simulink model "gm_uz_resolver_mech_revolution_float"  (R2021a)
settings: Solver=FixedStepDiscrete  StartTime=0.0  StopTime=3/f_mech*resolver_polepairs*2  RelTol=1e-3
undefined symbols (not defined in the file or in its folder): bitToRpsFactor_16bit, f_mech, machine_polepairs, resolver_polepairs, t_ADC
libraries: hdlmdlgenlib x9, simulink x1
settings Model: Creator=micha  LastModifiedBy=micha
settings SolverCC: AlgebraicLoopSolver=TrustRegion
settings DataIOCC: LimitDataPoints=on  SaveOutput=off  SaveTime=off
settings OptimizationCC: BlockReduction=off  ConditionallyExecuteInputs=off  DefaultParameterBehavior=Inlined  LifeSpan=inf
settings DebuggingCC: AlgebraicLoopMsg=error  InheritedTsInSrcMsg=none  SingleTaskRateTransMsg=error  AllowSymbolicDim=off  StrictBusMsg=ErrorOnBusTreatedAsVector  SFUnexpectedBacktrackingDiag=warning  SFNoUnconditionalDefaultTransitionDiag=warning  SFExecutionAtInitializationDiag=none  SFMachineParentedDataDiag=warning  ArithmeticOperatorsInVariantConditions=warning
settings HardwareCC: ProdBitPerPointer=32  ProdBitPerSizeT=32  ProdBitPerPtrDiffT=32  ProdLargestAtomicFloat=None  ProdIntDivRoundTo=Undefined  ProdEndianess=Unspecified  ProdWordSize=32  ProdHWDeviceType=ASIC/FPGA->ASIC/FPGA  ProdEqTarget=off
settings SFSimCC: SimUseLocalCustomCode=off  CustomCodeUndefinedFunction=UseInterfaceOnly
settings RTWCC: RTWUseLocalCustomCode=off
settings CodeAppCC: StateflowObjectComments=on
settings GRTTargetCC: TargetLangStandard=C89/C90 (ANSI)
settings ConfigComp: CovScope=ReferencedModels  CovMetricSettings=dw  CovSaveCumulativeToWorkspaceVar=on  CovSaveSingleToWorkspaceVar=on  CovExternalEMLEnable=off  CovSFcnEnable=off

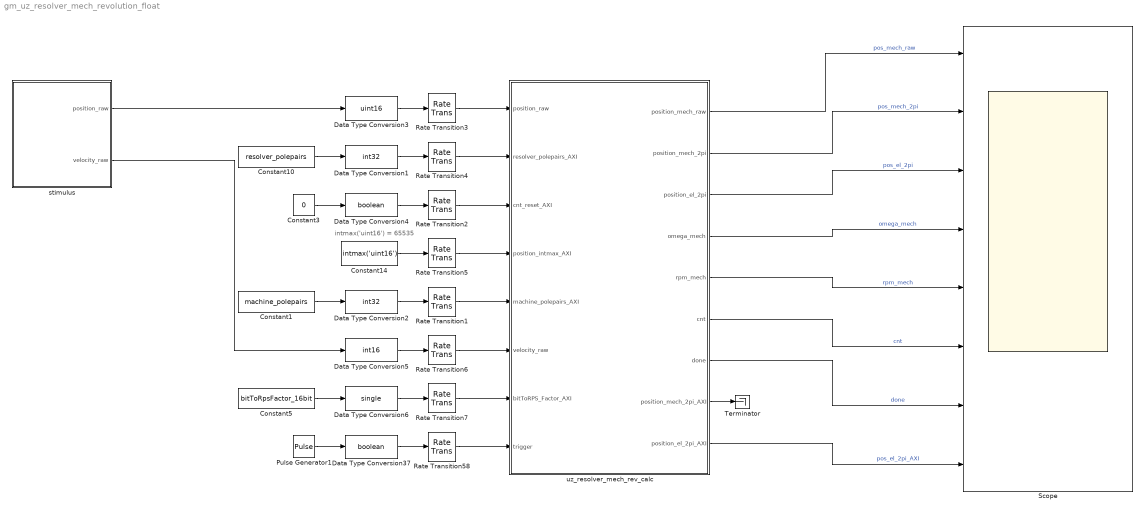
== system gm_uz_resolver_mech_revolution_float ==
  note: intmax('uint16') = 65535
  Constant1 : Constant  Value=machine_polepairs
  Constant10 : Constant  Value=resolver_polepairs
  Constant14 : Constant  Value=intmax('uint16')  OutDataTypeStr=int32  SampleTime=-1
  Constant3 : Constant  Value=0
  Constant5 : Constant  Value=bitToRpsFactor_16bit  SampleTime=-1
  Data Type Conversion1 : DataTypeConversion  OutDataTypeStr=int32
  Data Type Conversion2 : DataTypeConversion  OutDataTypeStr=int32
  Data Type Conversion3 : DataTypeConversion  OutDataTypeStr=uint16
  Data Type Conversion37 : DataTypeConversion  OutDataTypeStr=boolean
  Data Type Conversion4 : DataTypeConversion  OutDataTypeStr=boolean
  Data Type Conversion5 : DataTypeConversion  OutDataTypeStr=int16
  Data Type Conversion6 : DataTypeConversion  OutDataTypeStr=single
  Pulse Generator1 : DiscretePulseGenerator  PulseType=Time based  Period=t_ADC  PulseWidth=5
  Rate Transition{1..7,58} (8 alike) : RateTransition  OutPortSampleTime=t_clock
  Scope : Scope  NumInputPorts=8
  Terminator : Terminator
  stimulus : Subsystem
  uz_resolver_mech_rev_calc : Subsystem  TreatAsAtomicUnit=on
  wires:
  uz_resolver_mech_rev_calc/8(position_mech_2pi_AXI) -> Terminator/1
  uz_resolver_mech_rev_calc/9(position_el_2pi_AXI) -> Scope/8  "pos_el_2pi_AXI"
  uz_resolver_mech_rev_calc/5(rpm_mech) -> Scope/5  "rpm_mech"
  uz_resolver_mech_rev_calc/4(omega_mech) -> Scope/4  "omega_mech"
  Constant5/1 -> Data Type Conversion6/1
  Data Type Conversion6/1 -> Rate Transition7/1
  Rate Transition7/1 -> uz_resolver_mech_rev_calc/7(bitToRPS_Factor_AXI)
  stimulus/2(velocity_raw) -> Data Type Conversion5/1
  Rate Transition6/1 -> uz_resolver_mech_rev_calc/6(velocity_raw)
  Data Type Conversion5/1 -> Rate Transition6/1
  uz_resolver_mech_rev_calc/3(position_el_2pi) -> Scope/3  "pos_el_2pi"
  Rate Transition1/1 -> uz_resolver_mech_rev_calc/5(machine_polepairs_AXI)
  Constant1/1 -> Data Type Conversion2/1
  Data Type Conversion2/1 -> Rate Transition1/1
  stimulus/1(position_raw) -> Data Type Conversion3/1
  uz_resolver_mech_rev_calc/7(done) -> Scope/7  "done"
  uz_resolver_mech_rev_calc/6(cnt) -> Scope/6  "cnt"
  uz_resolver_mech_rev_calc/2(position_mech_2pi) -> Scope/2  "pos_mech_2pi"
  uz_resolver_mech_rev_calc/1(position_mech_raw) -> Scope/1  "pos_mech_raw"
  Data Type Conversion1/1 -> Rate Transition4/1
  Constant10/1 -> Data Type Conversion1/1
  Data Type Conversion3/1 -> Rate Transition3/1
  Rate Transition5/1 -> uz_resolver_mech_rev_calc/4(position_intmax_AXI)
  Constant14/1 -> Rate Transition5/1
  Rate Transition2/1 -> uz_resolver_mech_rev_calc/3(cnt_reset_AXI)
  Rate Transition3/1 -> uz_resolver_mech_rev_calc/1(position_raw)
  Rate Transition4/1 -> uz_resolver_mech_rev_calc/2(resolver_polepairs_AXI)
  Pulse Generator1/1 -> Data Type Conversion37/1
  Data Type Conversion37/1 -> Rate Transition58/1
  Data Type Conversion4/1 -> Rate Transition2/1
  Rate Transition58/1 -> uz_resolver_mech_rev_calc/8(trigger)
  Constant3/1 -> Data Type Conversion4/1

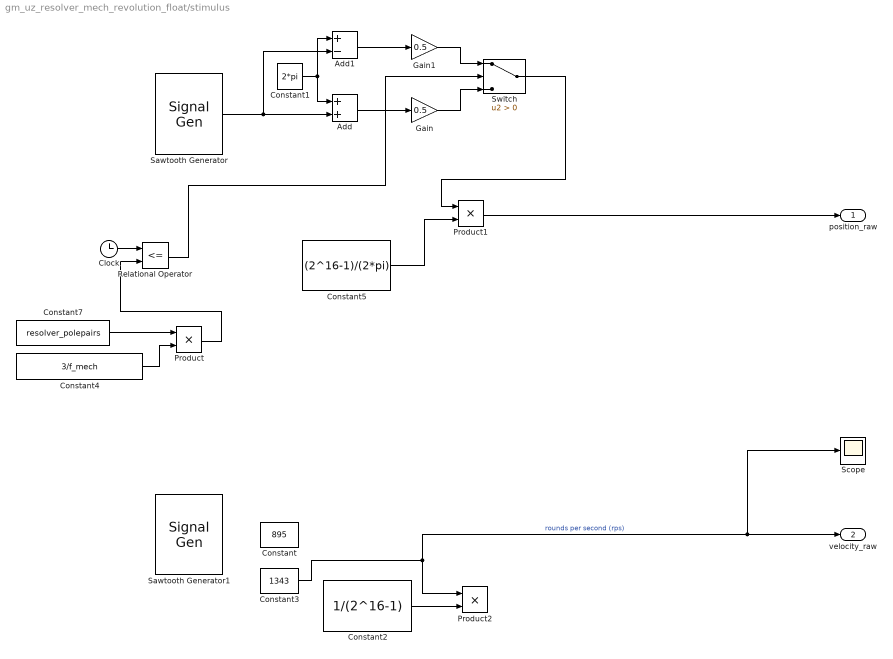
== system gm_uz_resolver_mech_revolution_float/stimulus ==
  Add : Sum
  Add1 : Sum  Inputs=+-
  Clock : Clock
  Constant : Constant  Value=895  SampleTime=-1
  Constant1 : Constant  Value=2*pi
  Constant2 : Constant  Value=1/(2^16-1)
  Constant3 : Constant  Value=1343  SampleTime=-1
  Constant4 : Constant  Value=3/f_mech
  Constant5 : Constant  Value=(2^16-1)/(2*pi)
  Constant7 : Constant  Value=resolver_polepairs
  Gain : Gain  Gain=0.5
  Gain1 : Gain  Gain=0.5
  Product : Product
  Product1 : Product
  Product2 : Product
  Relational Operator : RelationalOperator  Operator=<=  OutDataTypeStr=boolean  RndMeth=Simplest
  Sawtooth Generator : SignalGenerator  WaveForm=sawtooth  Amplitude=2*pi  Frequency=2*pi*f_mech  Units=rad/sec
  Sawtooth Generator1 : SignalGenerator  WaveForm=sawtooth  Frequency=2*pi*f_mech  Units=rad/sec
  Scope : Scope
  Switch : Switch  Criteria=u2 > Threshold
  position_raw : Outport
  velocity_raw : Outport  Port=2
  wires:
  Constant3/1 -> Product2/1, velocity_raw/1, Scope/1  "rounds per second (rps)"
  Constant2/1 -> Product2/2
  Product1/1 -> position_raw/1
  Relational Operator/1 -> Switch/2
  Constant7/1 -> Product/1
  Add/1 -> Gain/1
  Constant1/1 -> Add1/1, Add/1
  Gain1/1 -> Switch/1
  Add1/1 -> Gain1/1
  Switch/1 -> Product1/1
  Product/1 -> Relational Operator/2
  Constant5/1 -> Product1/2
  Gain/1 -> Switch/3
  Clock/1 -> Relational Operator/1
  Constant4/1 -> Product/2
  Sawtooth Generator/1 -> Add/2, Add1/2

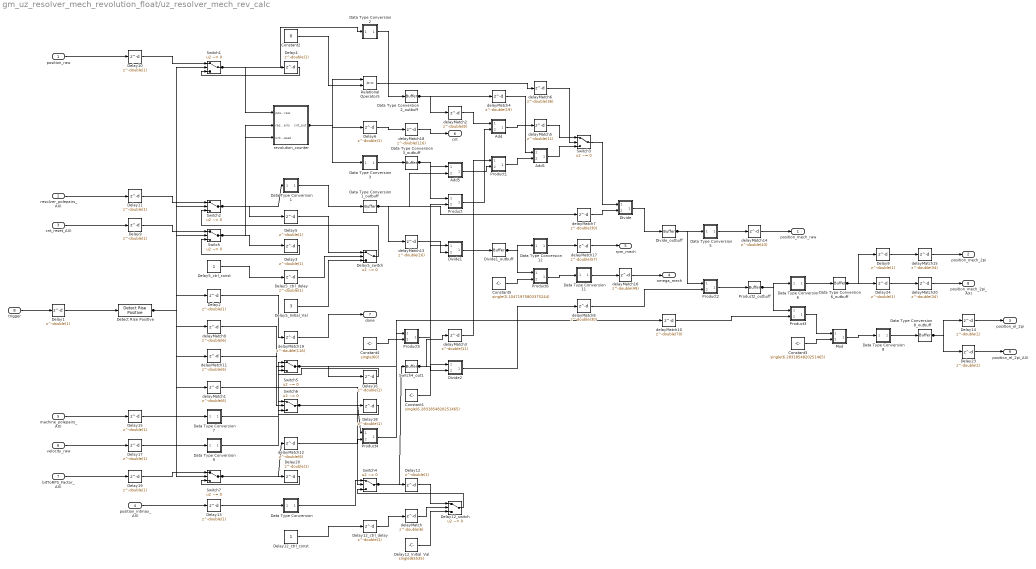
== system gm_uz_resolver_mech_revolution_float/uz_resolver_mech_rev_calc ==
  position_raw : Inport  OutDataTypeStr=uint16  PortDimensions=1  SampleTime=1e-08
  resolver_polepairs_AXI : Inport  Port=2  OutDataTypeStr=int32  PortDimensions=1  SampleTime=1e-08
  cnt_reset_AXI : Inport  Port=3  OutDataTypeStr=boolean  PortDimensions=1  SampleTime=1e-08
  position_intmax_AXI : Inport  Port=4  OutDataTypeStr=int32  PortDimensions=1  SampleTime=1e-08
  machine_polepairs_AXI : Inport  Port=5  OutDataTypeStr=int32  PortDimensions=1  SampleTime=1e-08
  velocity_raw : Inport  Port=6  OutDataTypeStr=int16  PortDimensions=1  SampleTime=1e-08
  bitToRPS_Factor_AXI : Inport  Port=7  OutDataTypeStr=single  PortDimensions=1  SampleTime=1e-08
  trigger : Inport  Port=8  OutDataTypeStr=boolean  PortDimensions=1  SampleTime=1e-08
  Add : Subsystem
      mask Display: disp('NFP\nadd');
  Add1 : Subsystem
      mask Display: disp('NFP\nadd');
  Add5 : Subsystem
      mask Display: disp('NFP\nadd');
  Constant1 : Constant  Value=single(6.2831854820251465)  OutDataTypeStr=single  SampleTime=1e-08
  Constant2 : Constant  Value=0  OutDataTypeStr=int16  SampleTime=1e-08
  Constant3 : Constant  Value=single(6.2831854820251465)  OutDataTypeStr=single  SampleTime=1e-08
  Constant4 : Constant  Value=single(60)  OutDataTypeStr=single  SampleTime=1e-08
  Constant5 : Constant  Value=single(0.10471975803375244)  OutDataTypeStr=single  SampleTime=1e-08
  Data Type Conversion : Subsystem
      mask Display: disp('NFP\nconv');
  Data Type Conversion1 : Subsystem
      mask Display: disp('NFP\nconv');
  Data Type Conversion11 : Subsystem
      mask Display: disp('NFP\nconv');
  Data Type Conversion12 : Subsystem
      mask Display: disp('NFP\nconv');
  Data Type Conversion1_outbuff : hdlmdlgenlib/Buffer
      settings: SourceProductBaseCode=SL
  Data Type Conversion2 : Subsystem
      mask Display: disp('NFP\nconv');
  Data Type Conversion2_outbuff : hdlmdlgenlib/Buffer
      settings: SourceProductBaseCode=SL
  Data Type Conversion3 : Subsystem
      mask Display: disp('NFP\nconv');
  Data Type Conversion3_outbuff : hdlmdlgenlib/Buffer
      settings: SourceProductBaseCode=SL
  Data Type Conversion5 : Subsystem
      mask Display: disp('NFP\nconv');
  Data Type Conversion6 : Subsystem
      mask Display: disp('NFP\nconv');
  Data Type Conversion6_outbuff : hdlmdlgenlib/Buffer
      settings: SourceProductBaseCode=SL
  Data Type Conversion7 : Subsystem
      mask Display: disp('NFP\nconv');
  Data Type Conversion8 : Subsystem
      mask Display: disp('NFP\nconv');
  Data Type Conversion8_outbuff : hdlmdlgenlib/Buffer
      settings: SourceProductBaseCode=SL
  Data Type Conversion9 : Subsystem
      mask Display: disp('NFP\nconv');
  Delay{1..6,8..20,23..24} (21 alike) : Delay  DelayLength=double(1)  InitialCondition=0  SampleTime=1e-08
  Delay12_Initial_Val : Constant  Value=single(65535)  OutDataTypeStr=single  SampleTime=1e-08
  Delay12_ctrl_const : Constant  OutDataTypeStr=boolean  SampleTime=1e-08
  Delay12_ctrl_delay : Delay  DelayLength=double(1)  InitialCondition=0  SampleTime=1e-08
  Delay12_switch : Switch  Criteria=u2 ~= 0  Threshold=double(0)  OutDataTypeStr=single  SampleTime=1e-08
  Delay5_Initial_Val : Constant  Value=3  OutDataTypeStr=int32  SampleTime=1e-08
  Delay5_ctrl_const : Constant  OutDataTypeStr=boolean  SampleTime=1e-08
  Delay5_ctrl_delay : Delay  DelayLength=double(1)  InitialCondition=0  SampleTime=1e-08
  Delay5_switch : Switch  Criteria=u2 ~= 0  Threshold=double(0)  OutDataTypeStr=int32  SampleTime=1e-08
  Detect Rise Positive : simulink/Logic and Bit Operations/Detect Rise Positive  vinit=0  OutDataTypeStr=boolean
  Divide : Subsystem
      mask Display: disp('NFP\nmul');
  Divide1 : Subsystem
      mask Display: disp('NFP\nmul');
  Divide1_outbuff : hdlmdlgenlib/Buffer
      settings: SourceProductBaseCode=SL
  Divide2 : Subsystem
      mask Display: disp('NFP\nmul');
  Divide_outbuff : hdlmdlgenlib/Buffer
      settings: SourceProductBaseCode=SL
  Mod : Subsystem
      mask Display: disp('NFP\nmath2');
  Product : Subsystem
      mask Display: disp('NFP\nmul');
  Product1 : Subsystem
      mask Display: disp('NFP\nmul');
  Product2 : Subsystem
      mask Display: disp('NFP\nmul');
  Product2_outbuff : hdlmdlgenlib/Buffer
      settings: SourceProductBaseCode=SL
  Product3 : Subsystem
      mask Display: disp('NFP\nmul');
  Product4 : Subsystem
      mask Display: disp('NFP\nmul');
  Product5 : Subsystem
      mask Display: disp('NFP\nmul');
  Product6 : Subsystem
      mask Display: disp('NFP\nmul');
  Relational Operator5 : RelationalOperator  OutDataTypeStr=boolean  SampleTime=1e-08  RndMeth=Nearest
  Switch : Switch  Criteria=u2 ~= 0  Threshold=double(0)  OutDataTypeStr=boolean  SampleTime=1e-08
  Switch1 : Switch  Criteria=u2 ~= 0  Threshold=double(0)  OutDataTypeStr=uint16  SampleTime=1e-08
  Switch2 : Switch  Criteria=u2 ~= 0  Threshold=double(0)  OutDataTypeStr=int32  SampleTime=1e-08
  Switch{3..7} (5 alike) : Switch  Criteria=u2 ~= 0  Threshold=double(0)  OutDataTypeStr=single  SampleTime=1e-08
  Switch4_out1 : hdlmdlgenlib/Buffer
      settings: SourceProductBaseCode=SL
  delayMatch{,1,9,11..12} (5 alike) : Delay  DelayLength=double(6)  InitialCondition=0  SampleTime=1e-08
  delayMatch10 : Delay  DelayLength=double(70)  InitialCondition=0  SampleTime=1e-08
  delayMatch13 : Delay  DelayLength=double(16)  InitialCondition=0  SampleTime=1e-08
  delayMatch14 : Delay  DelayLength=double(43)  InitialCondition=0  SampleTime=1e-08
  delayMatch15 : Delay  DelayLength=double(34)  InitialCondition=0  SampleTime=1e-08
  delayMatch16 : Delay  DelayLength=double(49)  InitialCondition=0  SampleTime=1e-08
  delayMatch17 : Delay  DelayLength=double(57)  InitialCondition=0  SampleTime=1e-08
  delayMatch18 : Delay  DelayLength=double(116)  InitialCondition=0  SampleTime=1e-08
  delayMatch19 : Delay  DelayLength=double(116)  InitialCondition=0  SampleTime=1e-08
  delayMatch2 : Delay  DelayLength=double(8)  InitialCondition=0  SampleTime=1e-08
  delayMatch20 : Delay  DelayLength=double(34)  InitialCondition=0  SampleTime=1e-08
  delayMatch3 : Delay  DelayLength=double(11)  InitialCondition=0  SampleTime=1e-08
  delayMatch4 : Delay  DelayLength=double(19)  InitialCondition=0  SampleTime=1e-08
  delayMatch5 : Delay  DelayLength=double(11)  InitialCondition=0  SampleTime=1e-08
  delayMatch6 : Delay  DelayLength=double(36)  InitialCondition=0  SampleTime=1e-08
  delayMatch7 : Delay  DelayLength=double(30)  InitialCondition=0  SampleTime=1e-08
  delayMatch8 : Delay  DelayLength=double(30)  InitialCondition=0  SampleTime=1e-08
  revolution_counter : Subsystem
  position_mech_raw : Outport  SampleTime=1e-08  VectorParamsAs1DForOutWhenUnconnected=off
  position_mech_2pi : Outport  Port=2  SampleTime=1e-08  VectorParamsAs1DForOutWhenUnconnected=off
  position_el_2pi : Outport  Port=3  SampleTime=1e-08  VectorParamsAs1DForOutWhenUnconnected=off
  omega_mech : Outport  Port=4  SampleTime=1e-08  VectorParamsAs1DForOutWhenUnconnected=off
  rpm_mech : Outport  Port=5  SampleTime=1e-08  VectorParamsAs1DForOutWhenUnconnected=off
  cnt : Outport  Port=6  SampleTime=1e-08  VectorParamsAs1DForOutWhenUnconnected=off
  done : Outport  Port=7  SampleTime=1e-08  VectorParamsAs1DForOutWhenUnconnected=off
  position_mech_2pi_AXI : Outport  Port=8  SampleTime=1e-08  VectorParamsAs1DForOutWhenUnconnected=off
  position_el_2pi_AXI : Outport  Port=9  SampleTime=1e-08  VectorParamsAs1DForOutWhenUnconnected=off
  wires:
  position_raw/1 -> Delay10/1
  resolver_polepairs_AXI/1 -> Delay11/1
  cnt_reset_AXI/1 -> Delay9/1
  position_intmax_AXI/1 -> Delay13/1
  machine_polepairs_AXI/1 -> Delay15/1
  velocity_raw/1 -> Delay17/1
  bitToRPS_Factor_AXI/1 -> Delay19/1
  trigger/1 -> Delay1/1
  delayMatch5/1 -> Switch3/1
  Constant1/1 -> Divide2/1(In1)
  Constant2/1 -> Relational Operator5/2
  Constant3/1 -> Mod/2(In2)
  Constant4/1 -> Product5/2(In2)
  Constant5/1 -> Product6/2(In2)
  delayMatch7/1 -> Divide/2(In2)
  delayMatch16/1 -> omega_mech/1
  delayMatch17/1 -> rpm_mech/1
  delayMatch2/1 -> Add/1(In1)
  Data Type Conversion3_outbuff/1 -> Product/1(In1), Add5/1(In1)
  delayMatch14/1 -> position_mech_raw/1
  Data Type Conversion6_outbuff/1 -> Delay8/1, Delay24/1
  Data Type Conversion8_outbuff/1 -> Delay23/1, Delay14/1
  Delay1/1 -> Detect Rise Positive/1
  Delay10/1 -> Switch1/1
  Delay11/1 -> Switch2/1
  Delay13/1 -> Data Type Conversion/1(In1)
  Delay14/1 -> position_el_2pi/1
  Delay15/1 -> Data Type Conversion7/1(In1)
  Delay17/1 -> Data Type Conversion9/1(In1)
  Delay19/1 -> Switch7/1
  delayMatch19/1 -> done/1
  Delay23/1 -> position_el_2pi_AXI/1
  delayMatch20/1 -> position_mech_2pi_AXI/1
  delayMatch18/1 -> cnt/1
  delayMatch15/1 -> position_mech_2pi/1
  Delay9/1 -> Switch/1
  delayMatch1/1 -> Switch4/2
  Divide_outbuff/1 -> Product2/1(In1), Data Type Conversion5/1(In1)
  Divide1_outbuff/1 -> Product6/1(In1), Data Type Conversion12/1(In1)
  delayMatch8/1 -> Product2/2(In2)
  Product2_outbuff/1 -> Product3/1(In1), Data Type Conversion6/1(In1)
  delayMatch6/1 -> Switch3/2
  Switch/1 -> revolution_counter/3(cnt_reset), Delay3/1
  Switch1/1 -> Data Type Conversion2/1(In1), revolution_counter/1(position_raw), Delay4/1
  Switch2/1 -> Data Type Conversion1/1(In1), revolution_counter/2(resolver_polepairs), Delay5/1
  Switch3/1 -> Divide/1(In1)
  delayMatch3/1 -> Product1/1(In1)
  delayMatch10/1 -> Product3/2(In2)
  delayMatch12/1 -> Product4/2(In2)
  revolution_counter/1(cnt_out) -> Data Type Conversion3/1(In1), Relational Operator5/1, Delay6/1
  Delay12_Initial_Val/1 -> Delay12_switch/3
  Delay12_ctrl_const/1 -> Delay12_ctrl_delay/1
  delayMatch/1 -> Delay12_switch/2
  Delay5_Initial_Val/1 -> Delay5_switch/3
  Delay5_ctrl_const/1 -> Delay5_ctrl_delay/1
  Delay5_ctrl_delay/1 -> Delay5_switch/2
  Add/1(Out1) -> delayMatch5/1
  Add1/1(Out1) -> Switch3/3
  Add5/1(Out1) -> Product1/2(In2)
  Data Type Conversion/1(Out1) -> Switch4/1
  Data Type Conversion1/1(Out1) -> Data Type Conversion1_outbuff/1
  Data Type Conversion11/1(Out1) -> delayMatch16/1
  Data Type Conversion12/1(Out1) -> delayMatch17/1
  Data Type Conversion2/1(Out1) -> Data Type Conversion2_outbuff/1
  Data Type Conversion3/1(Out1) -> Data Type Conversion3_outbuff/1
  Data Type Conversion5/1(Out1) -> delayMatch14/1
  Data Type Conversion6/1(Out1) -> Data Type Conversion6_outbuff/1
  Data Type Conversion7/1(Out1) -> Switch5/1
  Data Type Conversion8/1(Out1) -> Data Type Conversion8_outbuff/1
  Data Type Conversion9/1(Out1) -> Switch6/1
  Divide/1(Out1) -> Divide_outbuff/1
  Divide1/1(Out1) -> Divide1_outbuff/1
  Divide2/1(Out1) -> delayMatch8/1
  Mod/1(Out1) -> Data Type Conversion8/1(In1)
  Product/1(Out1) -> Add/2(In2)
  Product1/1(Out1) -> Add1/2(In2)
  Product2/1(Out1) -> Product2_outbuff/1
  Product3/1(Out1) -> Mod/1(In1)
  Product4/1(Out1) -> Product5/1(In1)
  Product5/1(Out1) -> Divide1/1(In1)
  Product6/1(Out1) -> Data Type Conversion11/1(In1)
  Delay12_ctrl_delay/1 -> delayMatch/1
  delayMatch9/1 -> Switch5/2
  delayMatch4/1 -> Add1/1(In1)
  Switch4_out1/1 -> delayMatch3/1, Product/2(In2), Divide2/2(In2)
  Data Type Conversion2_outbuff/1 -> delayMatch4/1, delayMatch2/1
  Relational Operator5/1 -> delayMatch6/1
  delayMatch13/1 -> Divide1/2(In2)
  delayMatch11/1 -> Switch6/2
  Detect Rise Positive/1 -> delayMatch11/1, delayMatch9/1, delayMatch1/1, Delay2/1, Switch1/2, Switch2/2, Switch/2, Switch7/2
  Switch7/1 -> delayMatch12/1, Delay20/1
  Data Type Conversion1_outbuff/1 -> delayMatch13/1, delayMatch7/1, Add5/2(In2)
  Delay8/1 -> delayMatch15/1
  Delay6/1 -> delayMatch18/1
  Delay2/1 -> delayMatch19/1
  Delay24/1 -> delayMatch20/1
  Switch4/1 -> Switch4_out1/1, Delay12/1
  Switch5/1 -> delayMatch10/1, Delay16/1
  Switch6/1 -> Product4/1(In1), Delay18/1
  Delay4/1 -> Switch1/3
  Delay5/1 -> Delay5_switch/1
  Delay5_switch/1 -> Switch2/3
  Delay3/1 -> Switch/3
  Delay12/1 -> Delay12_switch/1
  Delay12_switch/1 -> Switch4/3
  Delay16/1 -> Switch5/3
  Delay18/1 -> Switch6/3
  Delay20/1 -> Switch7/3

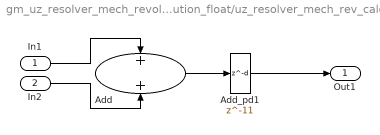
== system gm_uz_resolver_mech_revolution_float/uz_resolver_mech_rev_calc/Add ==
  In1 : Inport
  In2 : Inport  Port=2
  Add : Sum  OutDataTypeStr=single  SampleTime=1e-08
  Add_pd1 : Delay  DelayLength=11
  Out1 : Outport
  wires:
  In1/1 -> Add/1
  In2/1 -> Add/2
  Add/1 -> Add_pd1/1
  Add_pd1/1 -> Out1/1

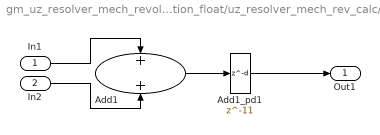
== system gm_uz_resolver_mech_revolution_float/uz_resolver_mech_rev_calc/Add1 ==
  In1 : Inport
  In2 : Inport  Port=2
  Add1 : Sum  OutDataTypeStr=single  SampleTime=1e-08
  Add1_pd1 : Delay  DelayLength=11
  Out1 : Outport
  wires:
  In1/1 -> Add1/1
  In2/1 -> Add1/2
  Add1/1 -> Add1_pd1/1
  Add1_pd1/1 -> Out1/1

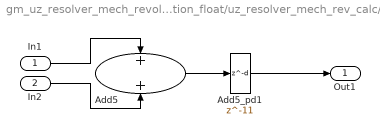
== system gm_uz_resolver_mech_revolution_float/uz_resolver_mech_rev_calc/Add5 ==
  In1 : Inport
  In2 : Inport  Port=2
  Add5 : Sum  OutDataTypeStr=single  SampleTime=1e-08
  Add5_pd1 : Delay  DelayLength=11
  Out1 : Outport
  wires:
  In1/1 -> Add5/1
  In2/1 -> Add5/2
  Add5/1 -> Add5_pd1/1
  Add5_pd1/1 -> Out1/1

== system gm_uz_resolver_mech_revolution_float/uz_resolver_mech_rev_calc/Data Type Conversion ==
  In1 : Inport
  Data Type Conversion : DataTypeConversion  OutDataTypeStr=single  SampleTime=1e-08
  Data Type Conversion_pd1 : Delay  DelayLength=6
  Out1 : Outport
  wires:
  In1/1 -> Data Type Conversion/1
  Data Type Conversion/1 -> Data Type Conversion_pd1/1
  Data Type Conversion_pd1/1 -> Out1/1

== system gm_uz_resolver_mech_revolution_float/uz_resolver_mech_rev_calc/Data Type Conversion1 ==
  In1 : Inport
  Data Type Conversion1 : DataTypeConversion  OutDataTypeStr=single  SampleTime=1e-08
  Data Type Conversion1_pd1 : Delay  DelayLength=6
  Out1 : Outport
  wires:
  In1/1 -> Data Type Conversion1/1
  Data Type Conversion1/1 -> Data Type Conversion1_pd1/1
  Data Type Conversion1_pd1/1 -> Out1/1

== system gm_uz_resolver_mech_revolution_float/uz_resolver_mech_rev_calc/Data Type Conversion11 ==
  In1 : Inport
  Data Type Conversion11 : DataTypeConversion  OutDataTypeStr=fixdt(1, 24, 11)  SampleTime=1e-08
  Data Type Conversion11_pd1 : Delay  DelayLength=6
  Out1 : Outport
  wires:
  In1/1 -> Data Type Conversion11/1
  Data Type Conversion11/1 -> Data Type Conversion11_pd1/1
  Data Type Conversion11_pd1/1 -> Out1/1

== system gm_uz_resolver_mech_revolution_float/uz_resolver_mech_rev_calc/Data Type Conversion12 ==
  In1 : Inport
  Data Type Conversion12 : DataTypeConversion  OutDataTypeStr=fixdt(1, 24, 11)  SampleTime=1e-08
  Data Type Conversion12_pd1 : Delay  DelayLength=6
  Out1 : Outport
  wires:
  In1/1 -> Data Type Conversion12/1
  Data Type Conversion12/1 -> Data Type Conversion12_pd1/1
  Data Type Conversion12_pd1/1 -> Out1/1

== system gm_uz_resolver_mech_revolution_float/uz_resolver_mech_rev_calc/Data Type Conversion2 ==
  In1 : Inport
  Data Type Conversion2 : DataTypeConversion  OutDataTypeStr=single  SampleTime=1e-08
  Data Type Conversion2_pd1 : Delay  DelayLength=6
  Out1 : Outport
  wires:
  In1/1 -> Data Type Conversion2/1
  Data Type Conversion2/1 -> Data Type Conversion2_pd1/1
  Data Type Conversion2_pd1/1 -> Out1/1

== system gm_uz_resolver_mech_revolution_float/uz_resolver_mech_rev_calc/Data Type Conversion3 ==
  In1 : Inport
  Data Type Conversion3 : DataTypeConversion  OutDataTypeStr=single  SampleTime=1e-08
  Data Type Conversion3_pd1 : Delay  DelayLength=6
  Out1 : Outport
  wires:
  In1/1 -> Data Type Conversion3/1
  Data Type Conversion3/1 -> Data Type Conversion3_pd1/1
  Data Type Conversion3_pd1/1 -> Out1/1

== system gm_uz_resolver_mech_revolution_float/uz_resolver_mech_rev_calc/Data Type Conversion5 ==
  In1 : Inport
  Data Type Conversion5 : DataTypeConversion  OutDataTypeStr=uint16  SampleTime=1e-08
  Data Type Conversion5_pd1 : Delay  DelayLength=6
  Out1 : Outport
  wires:
  In1/1 -> Data Type Conversion5/1
  Data Type Conversion5/1 -> Data Type Conversion5_pd1/1
  Data Type Conversion5_pd1/1 -> Out1/1

== system gm_uz_resolver_mech_revolution_float/uz_resolver_mech_rev_calc/Data Type Conversion6 ==
  In1 : Inport
  Data Type Conversion6 : DataTypeConversion  OutDataTypeStr=fixdt(1, 27, 20)  SampleTime=1e-08
  Data Type Conversion6_pd1 : Delay  DelayLength=6
  Out1 : Outport
  wires:
  In1/1 -> Data Type Conversion6/1
  Data Type Conversion6/1 -> Data Type Conversion6_pd1/1
  Data Type Conversion6_pd1/1 -> Out1/1

== system gm_uz_resolver_mech_revolution_float/uz_resolver_mech_rev_calc/Data Type Conversion7 ==
  In1 : Inport
  Data Type Conversion7 : DataTypeConversion  OutDataTypeStr=single  SampleTime=1e-08
  Data Type Conversion7_pd1 : Delay  DelayLength=6
  Out1 : Outport
  wires:
  In1/1 -> Data Type Conversion7/1
  Data Type Conversion7/1 -> Data Type Conversion7_pd1/1
  Data Type Conversion7_pd1/1 -> Out1/1

== system gm_uz_resolver_mech_revolution_float/uz_resolver_mech_rev_calc/Data Type Conversion8 ==
  In1 : Inport
  Data Type Conversion8 : DataTypeConversion  OutDataTypeStr=fixdt(1, 27, 20)  SampleTime=1e-08
  Data Type Conversion8_pd1 : Delay  DelayLength=6
  Out1 : Outport
  wires:
  In1/1 -> Data Type Conversion8/1
  Data Type Conversion8/1 -> Data Type Conversion8_pd1/1
  Data Type Conversion8_pd1/1 -> Out1/1

== system gm_uz_resolver_mech_revolution_float/uz_resolver_mech_rev_calc/Data Type Conversion9 ==
  In1 : Inport
  Data Type Conversion9 : DataTypeConversion  OutDataTypeStr=single  SampleTime=1e-08
  Data Type Conversion9_pd1 : Delay  DelayLength=6
  Out1 : Outport
  wires:
  In1/1 -> Data Type Conversion9/1
  Data Type Conversion9/1 -> Data Type Conversion9_pd1/1
  Data Type Conversion9_pd1/1 -> Out1/1

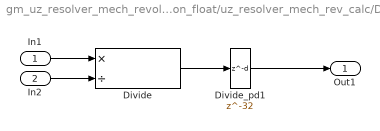
== system gm_uz_resolver_mech_revolution_float/uz_resolver_mech_rev_calc/Divide ==
  In1 : Inport
  In2 : Inport  Port=2
  Divide : Product  Inputs=*/  OutDataTypeStr=single  RndMeth=Simplest  SaturateOnIntegerOverflow=on  SampleTime=1e-08
  Divide_pd1 : Delay  DelayLength=32
  Out1 : Outport
  wires:
  In1/1 -> Divide/1
  In2/1 -> Divide/2
  Divide/1 -> Divide_pd1/1
  Divide_pd1/1 -> Out1/1

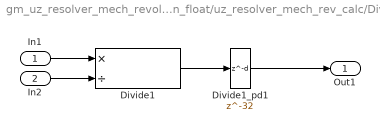
== system gm_uz_resolver_mech_revolution_float/uz_resolver_mech_rev_calc/Divide1 ==
  In1 : Inport
  In2 : Inport  Port=2
  Divide1 : Product  Inputs=*/  OutDataTypeStr=single  SampleTime=1e-08
  Divide1_pd1 : Delay  DelayLength=32
  Out1 : Outport
  wires:
  In1/1 -> Divide1/1
  In2/1 -> Divide1/2
  Divide1/1 -> Divide1_pd1/1
  Divide1_pd1/1 -> Out1/1

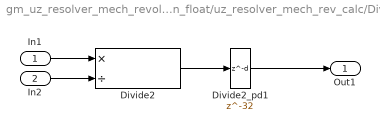
== system gm_uz_resolver_mech_revolution_float/uz_resolver_mech_rev_calc/Divide2 ==
  In1 : Inport
  In2 : Inport  Port=2
  Divide2 : Product  Inputs=*/  OutDataTypeStr=single  RndMeth=Simplest  SaturateOnIntegerOverflow=on  SampleTime=1e-08
  Divide2_pd1 : Delay  DelayLength=32
  Out1 : Outport
  wires:
  In1/1 -> Divide2/1
  In2/1 -> Divide2/2
  Divide2/1 -> Divide2_pd1/1
  Divide2_pd1/1 -> Out1/1

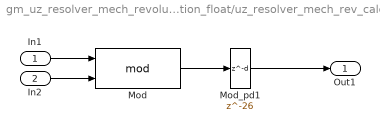
== system gm_uz_resolver_mech_revolution_float/uz_resolver_mech_rev_calc/Mod ==
  In1 : Inport
  In2 : Inport  Port=2
  Mod : Math  Operator=mod  SampleTime=1e-08  SaturateOnIntegerOverflow=on
  Mod_pd1 : Delay  DelayLength=26
  Out1 : Outport
  wires:
  In1/1 -> Mod/1
  In2/1 -> Mod/2
  Mod/1 -> Mod_pd1/1
  Mod_pd1/1 -> Out1/1

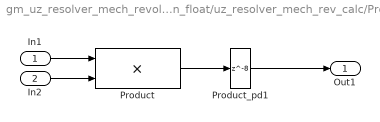
== system gm_uz_resolver_mech_revolution_float/uz_resolver_mech_rev_calc/Product ==
  In1 : Inport
  In2 : Inport  Port=2
  Product : Product  Inputs=**  OutDataTypeStr=single  SampleTime=1e-08
  Product_pd1 : Delay  DelayLength=8
  Out1 : Outport
  wires:
  In1/1 -> Product/1
  In2/1 -> Product/2
  Product/1 -> Product_pd1/1
  Product_pd1/1 -> Out1/1

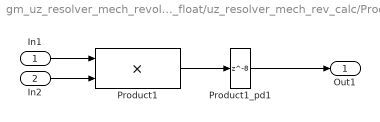
== system gm_uz_resolver_mech_revolution_float/uz_resolver_mech_rev_calc/Product1 ==
  In1 : Inport
  In2 : Inport  Port=2
  Product1 : Product  Inputs=**  OutDataTypeStr=single  SampleTime=1e-08
  Product1_pd1 : Delay  DelayLength=8
  Out1 : Outport
  wires:
  In1/1 -> Product1/1
  In2/1 -> Product1/2
  Product1/1 -> Product1_pd1/1
  Product1_pd1/1 -> Out1/1

== system gm_uz_resolver_mech_revolution_float/uz_resolver_mech_rev_calc/Product2 ==
  In1 : Inport
  In2 : Inport  Port=2
  Product2 : Product  Inputs=**  OutDataTypeStr=single  SampleTime=1e-08
  Product2_pd1 : Delay  DelayLength=8
  Out1 : Outport
  wires:
  In1/1 -> Product2/1
  In2/1 -> Product2/2
  Product2/1 -> Product2_pd1/1
  Product2_pd1/1 -> Out1/1

== system gm_uz_resolver_mech_revolution_float/uz_resolver_mech_rev_calc/Product3 ==
  In1 : Inport
  In2 : Inport  Port=2
  Product3 : Product  Inputs=**  OutDataTypeStr=single  SampleTime=1e-08
  Product3_pd1 : Delay  DelayLength=8
  Out1 : Outport
  wires:
  In1/1 -> Product3/1
  In2/1 -> Product3/2
  Product3/1 -> Product3_pd1/1
  Product3_pd1/1 -> Out1/1

== system gm_uz_resolver_mech_revolution_float/uz_resolver_mech_rev_calc/Product4 ==
  In1 : Inport
  In2 : Inport  Port=2
  Product4 : Product  Inputs=**  OutDataTypeStr=single  SampleTime=1e-08
  Product4_pd1 : Delay  DelayLength=8
  Out1 : Outport
  wires:
  In1/1 -> Product4/1
  In2/1 -> Product4/2
  Product4/1 -> Product4_pd1/1
  Product4_pd1/1 -> Out1/1

== system gm_uz_resolver_mech_revolution_float/uz_resolver_mech_rev_calc/Product5 ==
  In1 : Inport
  In2 : Inport  Port=2
  Product5 : Product  Inputs=**  OutDataTypeStr=single  SampleTime=1e-08
  Product5_pd1 : Delay  DelayLength=8
  Out1 : Outport
  wires:
  In1/1 -> Product5/1
  In2/1 -> Product5/2
  Product5/1 -> Product5_pd1/1
  Product5_pd1/1 -> Out1/1

== system gm_uz_resolver_mech_revolution_float/uz_resolver_mech_rev_calc/Product6 ==
  In1 : Inport
  In2 : Inport  Port=2
  Product6 : Product  Inputs=**  OutDataTypeStr=single  SampleTime=1e-08
  Product6_pd1 : Delay  DelayLength=8
  Out1 : Outport
  wires:
  In1/1 -> Product6/1
  In2/1 -> Product6/2
  Product6/1 -> Product6_pd1/1
  Product6_pd1/1 -> Out1/1

== system gm_uz_resolver_mech_revolution_float/uz_resolver_mech_rev_calc/revolution_counter ==
  position_raw : Inport  OutDataTypeStr=uint16  PortDimensions=1  SampleTime=1e-08
  resolver_polepairs : Inport  Port=2  OutDataTypeStr=int32  PortDimensions=1  SampleTime=1e-08
  cnt_reset : Inport  Port=3  OutDataTypeStr=boolean  PortDimensions=1  SampleTime=1e-08
  revolution_counter : MATLAB Function  TreatAsAtomicUnit=on
  cnt_out : Outport  SampleTime=1e-08  VectorParamsAs1DForOutWhenUnconnected=off
  wires:
  revolution_counter/1(cnt_out) -> cnt_out/1
  position_raw/1 -> revolution_counter/1(position_raw)
  resolver_polepairs/1 -> revolution_counter/2(resolver_polepairs)
  cnt_reset/1 -> revolution_counter/3(cnt_reset)

== matlab function gm_uz_resolver_mech_revolution_float/uz_resolver_mech_rev_calc/revolution_counter/revolution_counter ==
  settings: fimath=fimath('RoundingMethod', 'Floor','OverflowAction', 'Wrap','ProductMode', 'FullPrecision', 'SumMode', 'FullPrecision')
  data: position_raw input; cnt_out output; resolver_polepairs input; cnt_reset input
function cnt_out  = fcn(position_raw, resolver_polepairs, cnt_reset)
%#codegen
persistent angle_mech_old;
if isempty(angle_mech_old)
    angle_mech_old = int32(0);
end

persistent cnt;
if isempty(cnt)
    cnt = int32(0);
end

if ((angle_mech_old-int32(position_raw)) > int32(60000))
    cnt = cnt+1;
elseif ((angle_mech_old-int32(position_raw)) < int32(-60000))
    cnt = cnt-1;
end

if (cnt > (resolver_polepairs-1) || cnt < -(resolver_polepairs-1))
    cnt = int32(0);
end

if (cnt_reset == true)
    cnt = int32(0);
end

angle_mech_old = int32(position_raw);
cnt_out = cnt;
end
